simulink model "AuE6610_Project_CV"  (R2025a)
settings: Solver=ode4  StartTime=0.0  StopTime=1874  FixedStep=0.1  RelTol=1e-3
values from neighbouring files (symbols this model uses):
  area_frontal = 2.18    [CV_Powertrain.m]    (also in EV_Powertrain.m; database.m)
  curb_weight = 1377    [CV_Powertrain.m]    (also in EV_Powertrain.m; database.m)
  drag_coefficient = 0.29    [CV_Powertrain.m]    (also in EV_Powertrain.m; database.m)
  eng =     [Engine_Data.mat]
  fdr = 4.21    [CV_Powertrain.m]    (also in EV_Powertrain.m; database.m)
  fdr_inertia = 0.02    [CV_Powertrain.m]    (also in EV_Powertrain.m; database.m)
  gear = [3.54, 1.91, 1.31, 0.97, 0.71, 0.62]    [CV_Powertrain.m]    (also in EV_Powertrain.m = 1.5; database.m)
  gear_no = [1, 2, 3, 4, 5, 6]    [CV_Powertrain.m]    (also in EV_Powertrain.m = 1; database.m = [1,2,3,4,5,6])
  gear_selected = zeros(length(peddle_position), length(speed))    [CV_Powertrain.m]    (also in database.m = zeros(length(iso_power), length(speed)))
  idle_rpm = 500    [CV_Powertrain.m]    (also in EV_Powertrain.m = 1; database.m)
  max_engine_power = max((rpm_engine_data(1,:) * (pi/30)) .* torque_engine_data(end,:))    [CV_Powertrain.m]    (also in database.m = max((rpm_engine_data(1,:) * ( pi /30)) .* torque_engine_data)
  peddle_position = 0.1:0.05:1    [CV_Powertrain.m]    (also in database.m)
  radius = 0.4318    [CV_Powertrain.m]    (also in EV_Powertrain.m; database.m)
  redline_rpm = 6800    [CV_Powertrain.m]    (also in EV_Powertrain.m = 11000; database.m)
  rho_air = 1.18    [CV_Powertrain.m]    (also in EV_Powertrain.m = 1.21; database.m)
  rolling_resistance_coefficient = 0.01    [CV_Powertrain.m]    (also in EV_Powertrain.m; database.m)
  rpm_reference_array = rpm_engine_data(1,:)    [CV_Powertrain.m]    (also in database.m)
  speed = 0:1:52    [CV_Powertrain.m]    (also in database.m = 1:1:52)
  torque_engine_data = zeros(n_pressure_points, n_rpm_points)    [CV_Powertrain.m]    (also in database.m = zeros(length(vol_eff_intake_pressure_array),length(rpm)))
  torque_max = torque_engine_data(end,:)    [CV_Powertrain.m]    (also in database.m)
  trans_inertia = 0.04    [CV_Powertrain.m]    (also in EV_Powertrain.m; database.m)
  wheel_inertia = 0.95    [CV_Powertrain.m]    (also in EV_Powertrain.m; database.m)
libraries: slpidlib x1, simulink x1
settings Model: Creator=Qilun Zhu  LastModifiedBy=abhi
settings SolverCC: ZeroCrossAlgorithm=Adaptive  AlgebraicLoopSolver=TrustRegion
settings DataIOCC: ReturnWorkspaceOutputs=off
settings DebuggingCC: UnconnectedInputMsg=warning  UnconnectedOutputMsg=warning  UnconnectedLineMsg=warning  ArithmeticOperatorsInVariantConditions=warning
settings ModelReferenceCC: EnableRefExpFcnMdlSchedulingChecks=on
settings SFSimCC: SimUseLocalCustomCode=off  CustomCodeUndefinedFunction=UseInterfaceOnly
settings RTWCC: RTWUseLocalCustomCode=off  GPUComputeCapability=3.5  DLArmComputeVersion=19.05
settings CodeAppCC: StateflowObjectComments=on
settings SimscapeCC: SimscapeNormalizeSystem=off

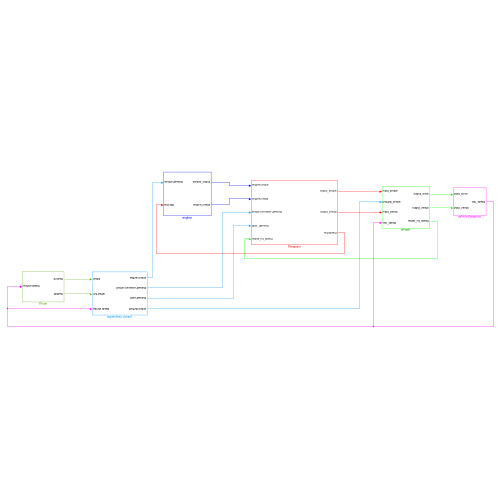
[thumbnail: Simulink's stored preview of the top-level diagram]
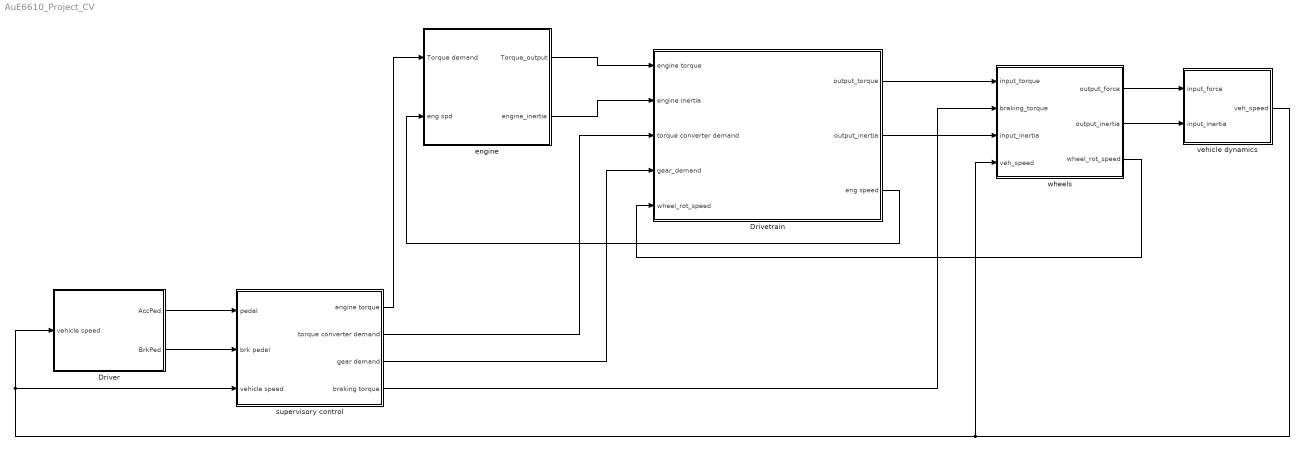
== system AuE6610_Project_CV ==
  Driver : Subsystem
  Drivetrain : Subsystem
  engine : Subsystem
  supervisory control : Subsystem
  vehicle dynamics : Subsystem
  wheels : Subsystem
  wires:
  supervisory control/1(engine torque) -> engine/1(Torque demand)
  wheels/1(output_force) -> vehicle dynamics/1(input_force)
  wheels/2(output_inertia) -> vehicle dynamics/2(input_inertia)
  supervisory control/4(braking torque) -> wheels/2(braking_torque)
  Driver/1(AccPed) -> supervisory control/1(" pedal")
  supervisory control/2(torque converter demand) -> Drivetrain/3(torque converter demand)
  supervisory control/3(gear demand) -> Drivetrain/4(gear_demand)
  engine/1(Torque_output) -> Drivetrain/1(engine torque)
  engine/2(engine_inertia) -> Drivetrain/2(engine inertia)
  wheels/3(wheel_rot_speed) -> Drivetrain/5(wheel_rot_speed)
  Drivetrain/1(output_torque) -> wheels/1(input_torque)
  Drivetrain/3(eng speed) -> engine/2(eng spd)
  Drivetrain/2(output_inertia) -> wheels/3(input_inertia)
  vehicle dynamics/1(veh_speed) -> Driver/1(vehicle speed), supervisory control/3(vehicle speed), wheels/4(veh_speed)
  Driver/2(BrkPed) -> supervisory control/2(" brk pedal")

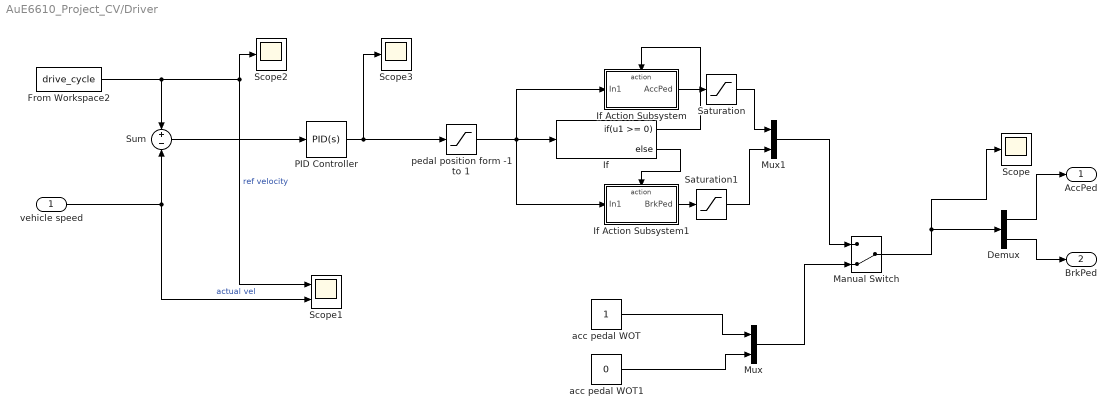
== system AuE6610_Project_CV/Driver ==
  vehicle speed : Inport
  Demux : Demux  Outputs=2
  From Workspace2 : FromWorkspace  VariableName=drive_cycle
  If : If  IfExpression=u1 >= 0
  If Action Subsystem : Subsystem  TreatAsAtomicUnit=on
  If Action Subsystem1 : Subsystem  TreatAsAtomicUnit=on
  Manual Switch : ManualSwitch  CurrentSetting=0
  Mux : Mux  Inputs=2
  Mux1 : Mux  Inputs=2
  PID Controller : slpidlib/PID Controller  Controller=PID  Form=Parallel  TimeDomain=Continuous-time  UseExternalTs=off  SampleTime=-1  IntegratorMethod=Forward Euler  FilterMethod=Forward Euler  ControllerParametersSource=internal  P=0.2  I=0.2  UseKiTs=off  D=0  UseExternalDerivativeSource=off  N=100  UseFilter=on  TunerSelectOption=Transfer Function Based (PID Tuner App)  InitialConditionSource=internal  InitialConditionForIntegrator=0  InitialConditionForFilter=0  DifferentiatorICPrevScaledInput=0  ExternalReset=none  TrackingMode=off  Kt=1  LimitOutput=off  SatLimitsSource=internal  UpperSaturationLimit=inf  LowerSaturationLimit=-inf  LinearizeAsGain=on  AntiWindupMode=none  Kb=1  LimitIntegrator=off  UpperIntegratorSaturationLimit=inf  LowerIntegratorSaturationLimit=-inf  POutMin=[]  POutMax=[]  IOutMin=[]  IOutMax=[]  DOutMin=[]  DOutMax=[]  NOutMin=[]  NOutMax=[]  SumOutMin=[]  SumOutMax=[]  SaturationOutMin=[]  SaturationOutMax=[]  PParamMin=[]  PParamMax=[]  IParamMin=[]  IParamMax=[]  DParamMin=[]  DParamMax=[]  NParamMin=[]  NParamMax=[]  KbParamMin=[]  KbParamMax=[]  KtParamMin=[]  KtParamMax=[]  KbOutMin=[]  KbOutMax=[]  KtOutMin=[]  KtOutMax=[]  IntegratorOutMin=[]  IntegratorOutMax=[]  FilterOutMin=[]  FilterOutMax=[]  SumI1OutMin=[]  SumI1OutMax=[]  SumI2OutMin=[]  SumI2OutMax=[]  SumI3OutMin=[]  SumI3OutMax=[]  SumI4OutMin=[]  SumI4OutMax=[]  SumDOutMin=[]  SumDOutMax=[]  DifferentiatorOutMin=[]  DifferentiatorOutMax=[]  FilterDiffOutCoefMin=[]  FilterDiffOutCoefMax=[]  ReciprocalOutMin=[]  ReciprocalOutMax=[]  SumDenOutMin=[]  SumDenOutMax=[]  SumNumOutMin=[]  SumNumOutMax=[]  DivideOutMin=[]  DivideOutMax=[]  UdiffTsProdOutMin=[]  UdiffTsProdOutMax=[]  NTsProdOutMin=[]  NTsProdOutMax=[]  UintegralTsProdOutMin=[]  UintegralTsProdOutMax=[]  UngainTsProdOutMin=[]  UngainTsProdOutMax=[]  ClampingZeroOutDataTypeStr=Inherit: Inherit via back propagation  ClampingZeroOutMin=[]  ClampingZeroOutMax=[]  FilterDenConstantOutDataTypeStr=Inherit: Inherit via back propagation  FilterDenConstantOutMin=[]  FilterDenConstantOutMax=[]  PCopyOutDataTypeStr=Inherit: Inherit via back propagation  PCopyOutMin=[]  PCopyOutMax=[]  NCopyOutDataTypeStr=Inherit: Inherit via back propagation  NCopyOutMin=[]  NCopyOutMax=[]  IntegratorContinuousStateAttributes=''  IntegratorStateMustResolveToSignalObject=off  IntegratorRTWStateStorageClass=Auto  FilterContinuousStateAttributes=''  FilterStateMustResolveToSignalObject=off  FilterRTWStateStorageClass=Auto  ParallelPVariant=InternalParameters  IdealPVariant=Disabled  IVariant=InternalParameters  DVariant=InternalParameters  IntegratorVariant=Continuous  SatVariant=Disabled  AWVariant=Passthrough  PCopyVariant=Disabled  TRVariant=Disabled  FdbkBlocksVariant=Forward  IdealPFdbkVariant=Disabled  SatFdbkVariant=Disabled  DerivativeFilterVariant=ContFilter  NVariant=InternalParameters  NCopyVariant=Disabled  FilterICVariant=InternalICsFilter  IntegratorICVariant=InternalICs  ExternalResetVariant=Disabled  TRSumVariant=Passthrough  SumFdbkVariant=Disabled  SumVariant=Sum_PID  TsampFilterVariant=InternalTs  TsampNgainVariant=Passthrough  TsampIntegralVariant=Disabled_SignalSpec  ExternalSaturationOutDataTypeStr=Inherit: Same as second input  DerivativeSourceVariant=ErrorSignal  PreIntVariant=InternalPreInt
  Saturation : Saturate  UpperLimit=1  LowerLimit=0
  Saturation1 : Saturate  UpperLimit=0  LowerLimit=-1
  Scope : Scope
      settings: ActiveDisplayYMinimum=-0.14734993314057482  ActiveDisplayYMaximum=0.25708356737728405
  Scope1 : Scope  NumInputPorts=2
      settings: ActiveDisplayYMinimum=-3.7898658117553516  ActiveDisplayYMaximum=28.746411818006802
  Scope2 : Scope
      settings: ActiveDisplayYMinimum=-1  ActiveDisplayYMaximum=1  DataLoggingVariableName=ScopeData2
  Scope3 : Scope
      settings: ActiveDisplayYMinimum=-1.9427647766660474  ActiveDisplayYMaximum=1.090909837606671  DataLoggingVariableName=ScopeData14
  Sum : Sum  Inputs=+-
  acc pedal WOT : Constant
  acc pedal WOT1 : Constant  Value=0
  pedal position form -1 to 1 : Saturate  UpperLimit=1  LowerLimit=-1  ZeroCross=off
  AccPed : Outport
  BrkPed : Outport  Port=2
  wires:
  Manual Switch/1 -> Demux/1, Scope/1
  If/1 -> If Action Subsystem/Action
  If/2 -> If Action Subsystem1/Action
  Sum/1 -> PID Controller/1
  pedal position form -1 to 1/1 -> If/1, If Action Subsystem1/1(In1), If Action Subsystem/1(In1)
  acc pedal WOT/1 -> Mux/1
  acc pedal WOT1/1 -> Mux/2
  Mux/1 -> Manual Switch/2
  Demux/1 -> AccPed/1
  Demux/2 -> BrkPed/1
  Mux1/1 -> Manual Switch/1
  From Workspace2/1 -> Scope2/1, Scope1/1, Sum/1  "ref velocity"
  vehicle speed/1 -> Scope1/2, Sum/2  "actual vel"
  PID Controller/1 -> Scope3/1, pedal position form -1 to 1/1
  If Action Subsystem/1(AccPed) -> Saturation/1
  Saturation/1 -> Mux1/1
  If Action Subsystem1/1(BrkPed) -> Saturation1/1
  Saturation1/1 -> Mux1/2

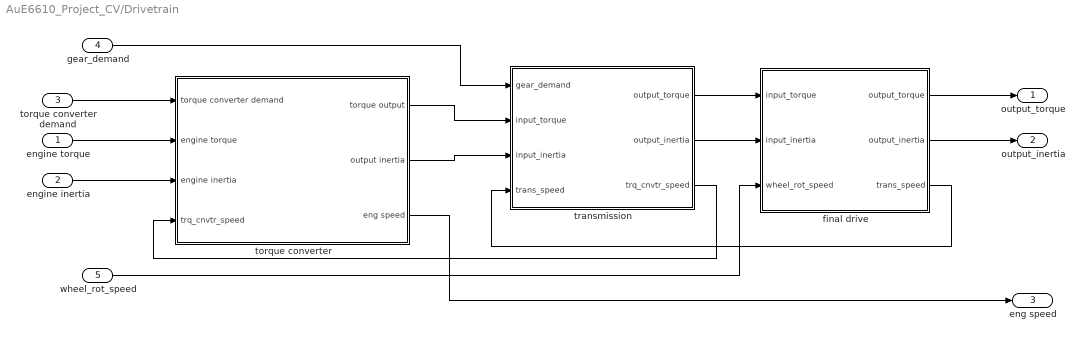
== system AuE6610_Project_CV/Drivetrain ==
  engine torque : Inport
  engine inertia : Inport  Port=2
  torque converter demand : Inport  Port=3
  gear_demand : Inport  Port=4
  wheel_rot_speed : Inport  Port=5
  final drive : Subsystem
      mask Display: image('C:\Users\bhatt\Desktop\driveline.jpg'); % Use "Edit Image" on toolstrip to change.
  torque converter : Subsystem
      mask Display: image('C:\Users\bhatt\Desktop\torque converter.jpg'); % Use "Edit Image" on toolstrip to change.
  transmission : Subsystem
      mask Display: image('C:\Users\bhatt\Desktop\gearbox.jpg'); % Use "Edit Image" on toolstrip to change.
  output_torque : Outport
  output_inertia : Outport  Port=2
  eng speed : Outport  Port=3
  wires:
  torque converter/3(eng speed) -> eng speed/1
  transmission/2(output_inertia) -> final drive/2(input_inertia)
  transmission/1(output_torque) -> final drive/1(input_torque)
  engine inertia/1 -> torque converter/3(engine inertia)
  torque converter/2(output inertia) -> transmission/3(input_inertia)
  final drive/3(trans_speed) -> transmission/4(trans_speed)
  torque converter/1(torque output) -> transmission/2(input_torque)
  transmission/3(trq_cnvtr_speed) -> torque converter/4(trq_cnvtr_speed)
  gear_demand/1 -> transmission/1(gear_demand)
  final drive/1(output_torque) -> output_torque/1
  engine torque/1 -> torque converter/2(engine torque)
  wheel_rot_speed/1 -> final drive/3(wheel_rot_speed)
  final drive/2(output_inertia) -> output_inertia/1
  torque converter demand/1 -> torque converter/1(torque converter demand)

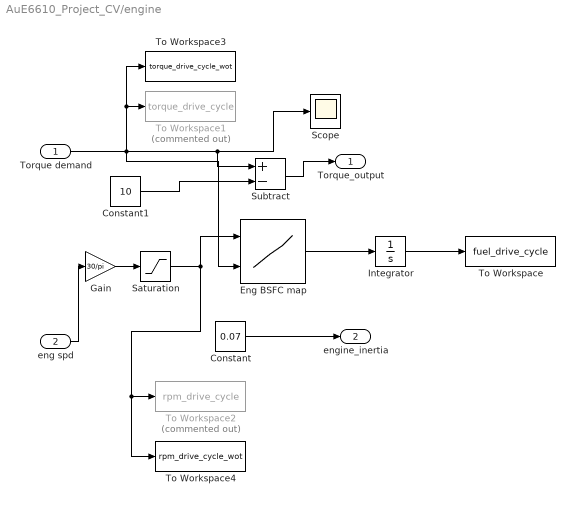
== system AuE6610_Project_CV/engine ==
  Torque demand : Inport
  eng spd : Inport  Port=2
  Constant : Constant  Value=0.07
  Constant1 : Constant  Value=10
  Eng BSFC map : Lookup_n-D  BreakpointsForDimension1=eng.BSFC.RPM  BreakpointsForDimension2=eng.BSFC.T  Table=eng.BSFC.fuel_rate  InternalRulePriority=Speed  RndMeth=Simplest
      settings: InputPortMap=u0,u1
  Gain : Gain  Gain=30/pi
  Integrator : Integrator
  Saturation : Saturate  UpperLimit=redline_rpm  LowerLimit=idle_rpm
  Scope : Scope
      settings: ActiveDisplayYMinimum=-16.725934018709687  ActiveDisplayYMaximum=150.53340616838722  DataLoggingVariableName=ScopeData3
  Subtract : Sum  Inputs=+-
  To Workspace : ToWorkspace  VariableName=fuel_drive_cycle  SampleTime=-1
  To Workspace1 : ToWorkspace  Commented=on  VariableName=torque_drive_cycle  SampleTime=-1
  To Workspace2 : ToWorkspace  Commented=on  VariableName=rpm_drive_cycle  SampleTime=-1
  To Workspace3 : ToWorkspace  VariableName=torque_drive_cycle_wot  SampleTime=-1
  To Workspace4 : ToWorkspace  VariableName=rpm_drive_cycle_wot  SampleTime=-1
  Torque_output : Outport
  engine_inertia : Outport  Port=2
  wires:
  eng spd/1 -> Gain/1
  Constant/1 -> engine_inertia/1
  Eng BSFC map/1 -> Integrator/1
  Torque demand/1 -> Subtract/1, Scope/1, To Workspace3/1, To Workspace1/1, Eng BSFC map/2
  Constant1/1 -> Subtract/2
  Subtract/1 -> Torque_output/1
  Gain/1 -> Saturation/1
  Saturation/1 -> To Workspace4/1, To Workspace2/1, Eng BSFC map/1
  Integrator/1 -> To Workspace/1

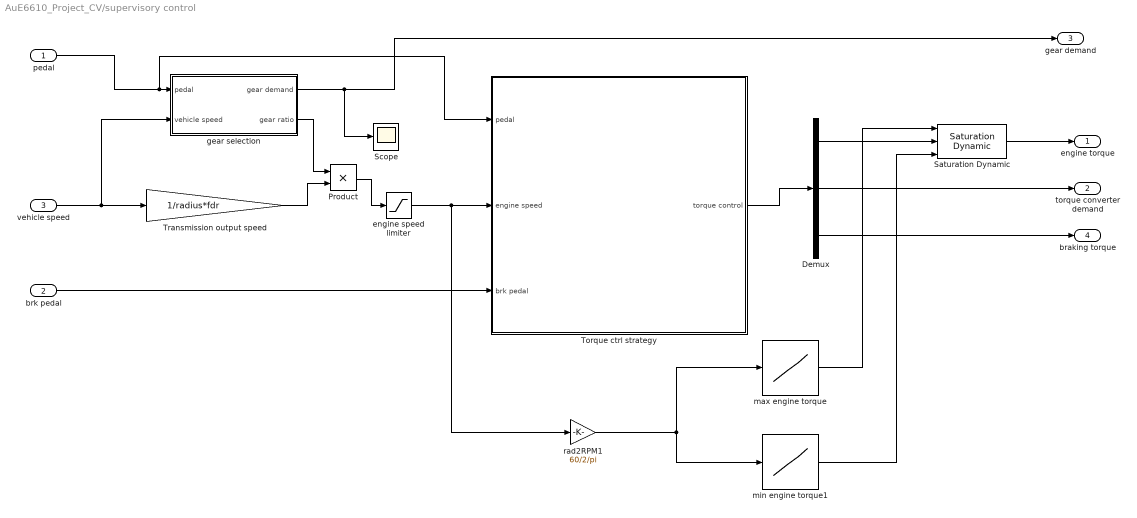
== system AuE6610_Project_CV/supervisory control ==
  " pedal" : Inport
  " brk pedal" : Inport  Port=2
  vehicle speed : Inport  Port=3
  Demux : Demux  Outputs=3
  Product : Product
  Saturation Dynamic : simulink/Discontinuities/Saturation Dynamic  OutMin=[]  OutMax=[]  OutDataTypeStr=Inherit: Same as second input  OutDataType=fixdt(1, 16)  OutScaling=2^-10  DoSatur=off
  Scope : Scope
      settings: ActiveDisplayYMinimum=-0.0099772185487898568  ActiveDisplayYMaximum=1.0167737074135261  DataLoggingVariableName=ScopeData16
  Torque ctrl strategy : Subsystem
  Transmission output speed : Gain  Gain=1/radius*fdr
  engine speed limiter : Saturate  UpperLimit=redline_rpm/60*2*pi  LowerLimit=idle_rpm/60*2*pi
  gear selection : Subsystem
  max engine torque : Lookup_n-D  NumberOfTableDimensions=1  BreakpointsForDimension1=rpm_reference_array  Table=torque_max  InternalRulePriority=Speed  RndMeth=Simplest
  min engine torque1 : Lookup_n-D  NumberOfTableDimensions=1  BreakpointsForDimension1=rpm_reference_array  Table=torque_engine_data(1,:)  InternalRulePriority=Speed  RndMeth=Simplest
  rad2RPM1 : Gain  Gain=60/2/pi
  engine torque : Outport
  torque converter demand : Outport  Port=2
  gear demand : Outport  Port=3
  braking torque : Outport  Port=4
  wires:
  max engine torque/1 -> Saturation Dynamic/1
  min engine torque1/1 -> Saturation Dynamic/3
  Demux/1 -> Saturation Dynamic/2
  Saturation Dynamic/1 -> engine torque/1
  Demux/2 -> torque converter demand/1
  Demux/3 -> braking torque/1
  Torque ctrl strategy/1(torque control) -> Demux/1
  rad2RPM1/1 -> max engine torque/1, min engine torque1/1
  engine speed limiter/1 -> rad2RPM1/1, Torque ctrl strategy/2(engine speed)
  Product/1 -> engine speed limiter/1
  " pedal"/1 -> Torque ctrl strategy/1(pedal), gear selection/1(pedal)
  vehicle speed/1 -> Transmission output speed/1, gear selection/2(vehicle speed)
  gear selection/2(gear ratio) -> Product/1
  Transmission output speed/1 -> Product/2
  gear selection/1(gear demand) -> Scope/1, gear demand/1
  " brk pedal"/1 -> Torque ctrl strategy/3(" brk pedal")

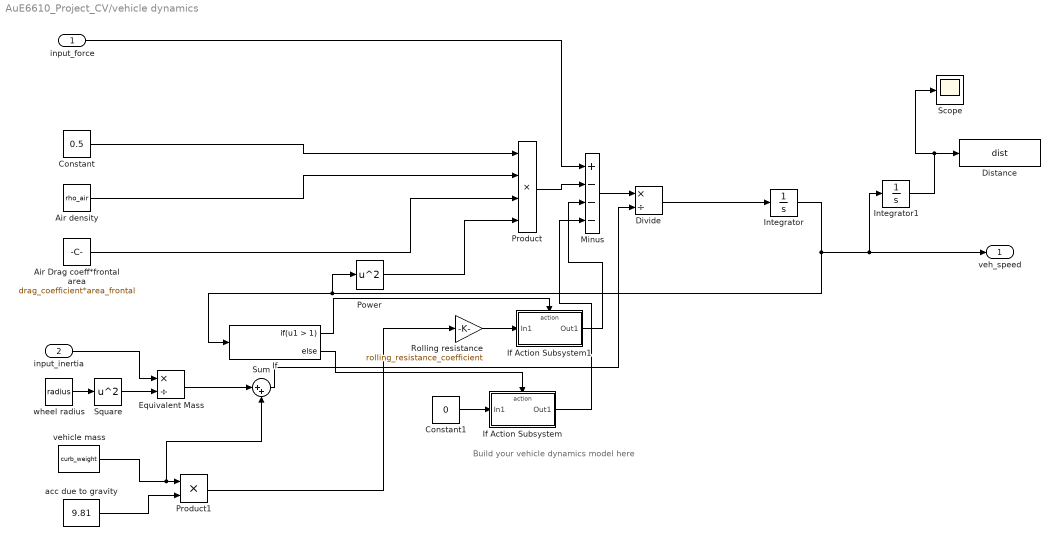
== system AuE6610_Project_CV/vehicle dynamics ==
  note: Build your vehicle dynamics model here
  input_force : Inport
  input_inertia : Inport  Port=2
  Air Drag coeff*frontal area : Constant  Value=drag_coefficient*area_frontal
  Air density : Constant  Value=rho_air
  Constant : Constant  Value=0.5
  Constant1 : Constant  Value=0
  Distance : ToWorkspace  VariableName=dist  SampleTime=-1
      settings: Save2DSignal=2-D array (concatenate along first dimension)
  Divide : Product  Inputs=*/
  Equivalent Mass : Product  Inputs=*/
  If : If  IfExpression=u1 > 1
  If Action Subsystem : Subsystem  TreatAsAtomicUnit=on
  If Action Subsystem1 : Subsystem  TreatAsAtomicUnit=on
  Integrator : Integrator
  Integrator1 : Integrator
  Minus : Sum  Inputs=+---
  Power : Math  Operator=square
  Product : Product  Inputs=4
  Product1 : Product
  "Rolling resistance " : Gain  Gain=rolling_resistance_coefficient
  Scope : Scope
      settings: ActiveDisplayYMinimum=-2221.2760263403779  ActiveDisplayYMaximum=19991.484237063407  DataLoggingVariableName=ScopeData5
  Square : Math  Operator=square
  Sum : Sum  Inputs=|++
  acc due to gravity : Constant  Value=9.81
  vehicle mass : Constant  Value=curb_weight
  wheel radius : Constant  Value=radius
  veh_speed : Outport
  wires:
  Product/1 -> Minus/2
  Integrator/1 -> If/1, Power/1, Integrator1/1, veh_speed/1
  If/1 -> If Action Subsystem1/Action
  If Action Subsystem1/1(Out1) -> Minus/3
  Divide/1 -> Integrator/1
  If Action Subsystem/1(Out1) -> Minus/4
  Minus/1 -> Divide/1
  "Rolling resistance "/1 -> If Action Subsystem1/1(In1)
  If/2 -> If Action Subsystem/Action
  input_force/1 -> Minus/1
  Constant/1 -> Product/1
  Air density/1 -> Product/2
  Air Drag coeff*frontal area/1 -> Product/3
  Power/1 -> Product/4
  vehicle mass/1 -> Sum/2, Product1/1
  acc due to gravity/1 -> Product1/2
  Product1/1 -> "Rolling resistance "/1
  Constant1/1 -> If Action Subsystem/1(In1)
  wheel radius/1 -> Square/1
  Square/1 -> Equivalent Mass/2
  input_inertia/1 -> Equivalent Mass/1
  Equivalent Mass/1 -> Sum/1
  Sum/1 -> Divide/2
  Integrator1/1 -> Scope/1, Distance/1

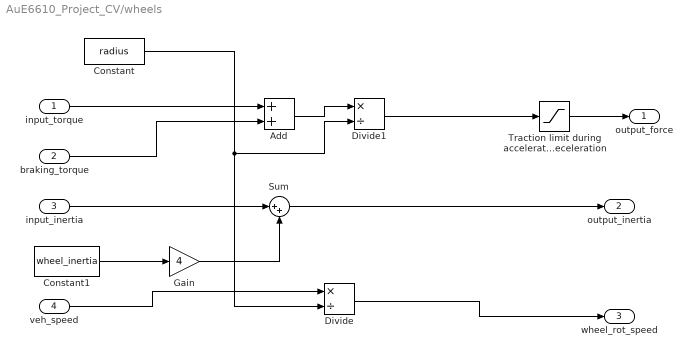
== system AuE6610_Project_CV/wheels ==
  input_torque : Inport
  braking_torque : Inport  Port=2
  input_inertia : Inport  Port=3
  veh_speed : Inport  Port=4
  Add : Sum
  Constant : Constant  Value=radius
  Constant1 : Constant  Value=wheel_inertia
  Divide : Product  Inputs=*/
  Divide1 : Product  Inputs=*/
  Gain : Gain  Gain=4
  Sum : Sum  Inputs=|++
  Traction limit during acceleration or deceleration : Saturate  UpperLimit=9740.781  LowerLimit=-9740.781
  output_force : Outport
  output_inertia : Outport  Port=2
  wheel_rot_speed : Outport  Port=3
  wires:
  Traction limit during acceleration or deceleration/1 -> output_force/1
  Constant/1 -> Divide1/2, Divide/2
  veh_speed/1 -> Divide/1
  Divide/1 -> wheel_rot_speed/1
  Constant1/1 -> Gain/1
  input_inertia/1 -> Sum/1
  Gain/1 -> Sum/2
  Sum/1 -> output_inertia/1
  input_torque/1 -> Add/1
  braking_torque/1 -> Add/2
  Add/1 -> Divide1/1
  Divide1/1 -> Traction limit during acceleration or deceleration/1

== system AuE6610_Project_CV/Driver/If Action Subsystem ==
  In1 : Inport
  Action Port : ActionPort  ActionPortLabel=if(u1 >= 0)
  AccPed : Outport
  wires:
  In1/1 -> AccPed/1

== system AuE6610_Project_CV/Driver/If Action Subsystem1 ==
  In1 : Inport
  Action Port : ActionPort  ActionPortLabel=else
  BrkPed : Outport
  wires:
  In1/1 -> BrkPed/1

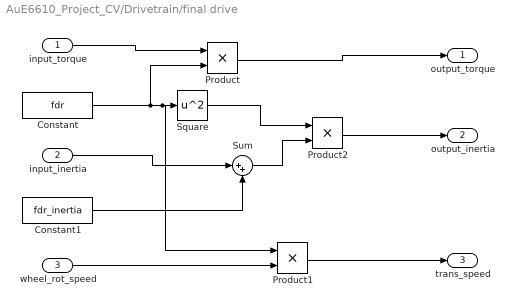
== system AuE6610_Project_CV/Drivetrain/final drive ==
  input_torque : Inport
  input_inertia : Inport  Port=2
  wheel_rot_speed : Inport  Port=3
  Constant : Constant  Value=fdr
  Constant1 : Constant  Value=fdr_inertia
  Product : Product
  Product1 : Product
  Product2 : Product
  Square : Math  Operator=square
  Sum : Sum  Inputs=|++
  output_torque : Outport
  output_inertia : Outport  Port=2
  trans_speed : Outport  Port=3
  wires:
  input_torque/1 -> Product/1
  Constant/1 -> Square/1, Product1/1, Product/2
  Product/1 -> output_torque/1
  input_inertia/1 -> Sum/1
  Constant1/1 -> Sum/2
  wheel_rot_speed/1 -> Product1/2
  Product1/1 -> trans_speed/1
  Product2/1 -> output_inertia/1
  Sum/1 -> Product2/2
  Square/1 -> Product2/1

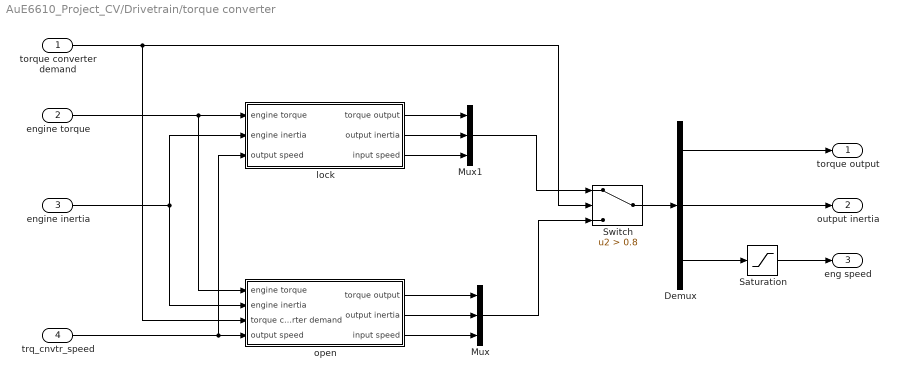
== system AuE6610_Project_CV/Drivetrain/torque converter ==
  torque converter demand : Inport
  engine torque : Inport  Port=2
  engine inertia : Inport  Port=3
  trq_cnvtr_speed : Inport  Port=4
  Demux : Demux  Outputs=3
  Mux : Mux  Inputs=3
  Mux1 : Mux  Inputs=3
  Saturation : Saturate  UpperLimit=6800/60*2*pi  LowerLimit=500/60*2*pi
  Switch : Switch  Criteria=u2 > Threshold  Threshold=0.8  SaturateOnIntegerOverflow=off  InputSameDT=off
  lock : Subsystem
  open : Subsystem
  torque output : Outport
  output inertia : Outport  Port=2
  eng speed : Outport  Port=3
  wires:
  engine torque/1 -> open/1(engine torque), lock/1(engine torque)
  engine inertia/1 -> open/2(engine inertia), lock/2(engine inertia)
  trq_cnvtr_speed/1 -> open/4(output speed), lock/3(output speed)
  open/1(torque output) -> Mux/1
  open/2(output inertia) -> Mux/2
  open/3(input speed) -> Mux/3
  lock/2(output inertia) -> Mux1/2
  lock/1(torque output) -> Mux1/1
  lock/3(input speed) -> Mux1/3
  torque converter demand/1 -> Switch/2, open/3(torque converter demand)
  Mux1/1 -> Switch/1
  Mux/1 -> Switch/3
  Switch/1 -> Demux/1
  Demux/1 -> torque output/1
  Demux/2 -> output inertia/1
  Demux/3 -> Saturation/1
  Saturation/1 -> eng speed/1

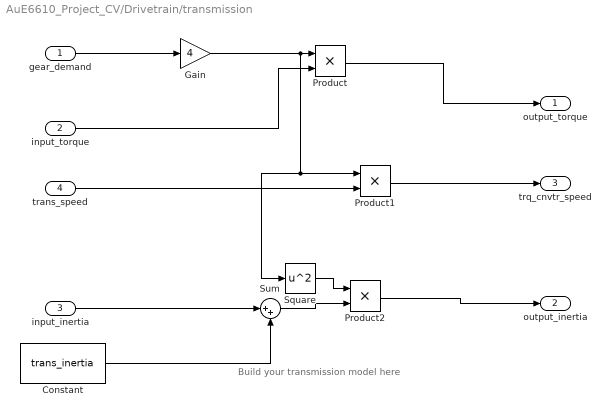
== system AuE6610_Project_CV/Drivetrain/transmission ==
  note: Build your transmission model here
  gear_demand : Inport
  input_torque : Inport  Port=2
  input_inertia : Inport  Port=3
  trans_speed : Inport  Port=4
  Constant : Constant  Value=trans_inertia
  Gain : Gain  Gain=4
  Product : Product
  Product1 : Product
  Product2 : Product
  Square : Math  Operator=square
  Sum : Sum  Inputs=|++
  output_torque : Outport
  output_inertia : Outport  Port=2
  trq_cnvtr_speed : Outport  Port=3
  wires:
  gear_demand/1 -> Gain/1
  Gain/1 -> Product1/1, Square/1, Product/1
  input_torque/1 -> Product/2
  Product/1 -> output_torque/1
  Constant/1 -> Sum/2
  input_inertia/1 -> Sum/1
  trans_speed/1 -> Product1/2
  Product1/1 -> trq_cnvtr_speed/1
  Square/1 -> Product2/1
  Sum/1 -> Product2/2
  Product2/1 -> output_inertia/1

== system AuE6610_Project_CV/supervisory control/Torque ctrl strategy ==
  pedal : Inport
  engine speed : Inport  Port=2
  " brk pedal" : Inport  Port=3
  Mux : Mux  Inputs=3
  Mux1 : Mux  Inputs=3
  Switch : Switch  Criteria=u2 > Threshold  ZeroCross=off  SaturateOnIntegerOverflow=off  InputSameDT=off
  accelerating : Subsystem
  decelerating : Subsystem
  torque control : Outport
  wires:
  engine speed/1 -> accelerating/2(engine speed), decelerating/1(engine speed)
  accelerating/1(engine torque) -> Mux/1
  accelerating/2(torque converter demand) -> Mux/2
  accelerating/3(braking torque) -> Mux/3
  decelerating/3(braking torque) -> Mux1/3
  decelerating/2(torque converter demand) -> Mux1/2
  decelerating/1(engine torque) -> Mux1/1
  Mux/1 -> Switch/1
  Mux1/1 -> Switch/3
  pedal/1 -> Switch/2, accelerating/1(acc pedal)
  Switch/1 -> torque control/1
  " brk pedal"/1 -> decelerating/2(brk pedal)

== system AuE6610_Project_CV/supervisory control/gear selection ==
  pedal : Inport
  vehicle speed : Inport  Port=2
  Maximum_Engine_Power : Constant  Commented=on  Value=max_engine_power
  gear map : Lookup_n-D  BreakpointsForDimension1=peddle_position  BreakpointsForDimension2=speed  Table=gear_selected  InterpMethod=Flat  InternalRulePriority=Speed  RndMeth=Simplest
      settings: InputPortMap=u0,u1
  selected gear ratio : Lookup_n-D  NumberOfTableDimensions=1  BreakpointsForDimension1=gear_no  Table=gear  InterpMethod=Flat  InternalRulePriority=Speed  RndMeth=Simplest
  gear demand : Outport
  gear ratio : Outport  Port=2
  wires:
  vehicle speed/1 -> gear map/2
  pedal/1 -> gear map/1
  gear map/1 -> gear demand/1, selected gear ratio/1
  selected gear ratio/1 -> gear ratio/1

== system AuE6610_Project_CV/vehicle dynamics/If Action Subsystem ==
  In1 : Inport
  Action Port : ActionPort  ActionPortLabel=else
  Out1 : Outport
  wires:
  In1/1 -> Out1/1

== system AuE6610_Project_CV/vehicle dynamics/If Action Subsystem1 ==
  In1 : Inport
  Action Port : ActionPort  ActionPortLabel=if(u1 > 1)
  Out1 : Outport
  wires:
  In1/1 -> Out1/1

== system AuE6610_Project_CV/Drivetrain/torque converter/lock ==
  engine torque : Inport
  engine inertia : Inport  Port=2
  output speed : Inport  Port=3
  torque output : Outport
  output inertia : Outport  Port=2
  input speed : Outport  Port=3
  wires:
  output speed/1 -> input speed/1
  engine torque/1 -> torque output/1
  engine inertia/1 -> output inertia/1

== system AuE6610_Project_CV/Drivetrain/torque converter/open ==
  engine torque : Inport
  engine inertia : Inport  Port=2
  torque converter demand : Inport  Port=3
  output speed : Inport  Port=4
  Constant : Constant  Value=0
  Constant1 : Constant  Value=0
  Divide : Product  Inputs=*/
  Integrator : Integrator  ExternalReset=falling  InitialConditionSource=external  InitialCondition=eng.rpm_idle/60*2*pi  ZeroCross=off
  torque output : Outport
  output inertia : Outport  Port=2
  input speed : Outport  Port=3
  wires:
  Constant/1 -> torque output/1
  engine torque/1 -> Divide/1
  engine inertia/1 -> Divide/2
  Divide/1 -> Integrator/1
  Integrator/1 -> input speed/1
  Constant1/1 -> output inertia/1
  torque converter demand/1 -> Integrator/2
  output speed/1 -> Integrator/3

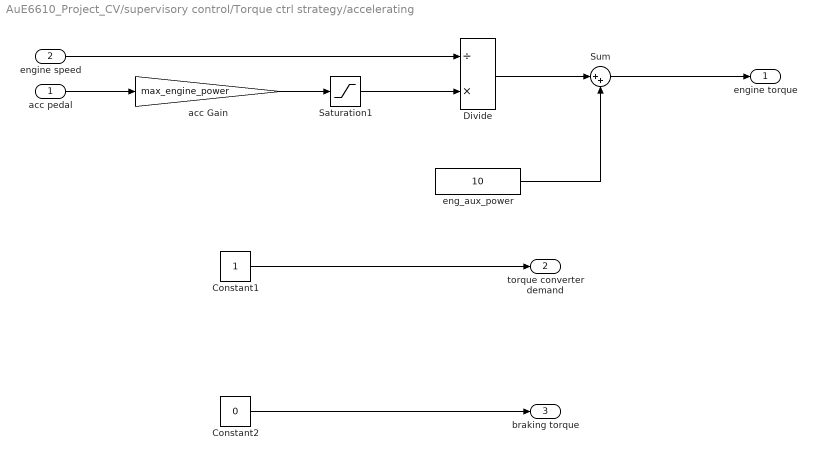
== system AuE6610_Project_CV/supervisory control/Torque ctrl strategy/accelerating ==
  acc pedal : Inport
  engine speed : Inport  Port=2
  Constant1 : Constant
  Constant2 : Constant  Value=0
  Divide : Product  Inputs=/*
  Saturation1 : Saturate  UpperLimit=max_engine_power  LowerLimit=0  ZeroCross=off
  Sum : Sum  Inputs=|++
  acc Gain : Gain  Gain=max_engine_power
  eng_aux_power : Constant  Value=10
  engine torque : Outport
  torque converter demand : Outport  Port=2
  braking torque : Outport  Port=3
  wires:
  engine speed/1 -> Divide/1
  eng_aux_power/1 -> Sum/2
  Divide/1 -> Sum/1
  Sum/1 -> engine torque/1
  Constant1/1 -> torque converter demand/1
  Constant2/1 -> braking torque/1
  acc Gain/1 -> Saturation1/1
  acc pedal/1 -> acc Gain/1
  Saturation1/1 -> Divide/2

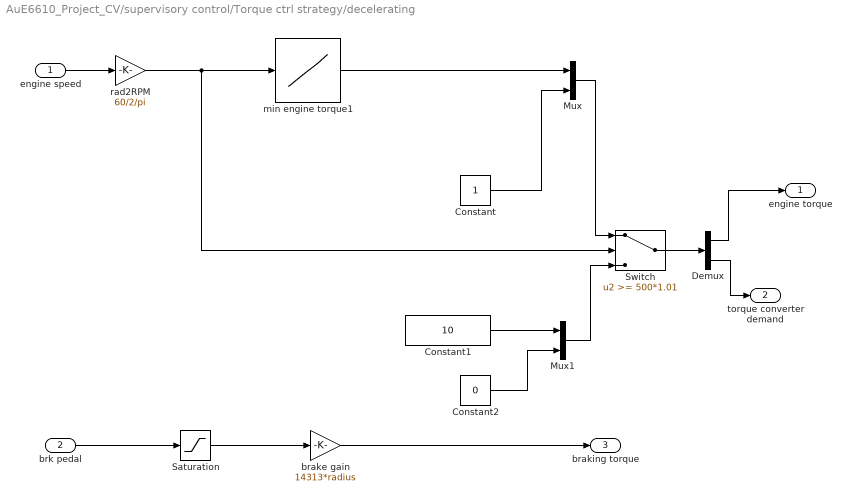
== system AuE6610_Project_CV/supervisory control/Torque ctrl strategy/decelerating ==
  engine speed : Inport
  brk pedal : Inport  Port=2
  Constant : Constant
  Constant1 : Constant  Value=10
  Constant2 : Constant  Value=0
  Demux : Demux  Outputs=2
  Mux : Mux  Inputs=2
  Mux1 : Mux  Inputs=2
  Saturation : Saturate  UpperLimit=0  LowerLimit=-1
  Switch : Switch  Threshold=500*1.01  ZeroCross=off  SaturateOnIntegerOverflow=off  InputSameDT=off
  brake gain : Gain  Gain=14313*radius
  min engine torque1 : Lookup_n-D  NumberOfTableDimensions=1  BreakpointsForDimension1=eng.T_max.RPM  Table=eng.T_min.T_min  InternalRulePriority=Speed  RndMeth=Simplest
  rad2RPM : Gain  Gain=60/2/pi
  engine torque : Outport
  torque converter demand : Outport  Port=2
  braking torque : Outport  Port=3
  wires:
  engine speed/1 -> rad2RPM/1
  rad2RPM/1 -> Switch/2, min engine torque1/1
  min engine torque1/1 -> Mux/1
  Constant/1 -> Mux/2
  Mux/1 -> Switch/1
  Constant1/1 -> Mux1/1
  Constant2/1 -> Mux1/2
  Mux1/1 -> Switch/3
  Switch/1 -> Demux/1
  Demux/1 -> engine torque/1
  Demux/2 -> torque converter demand/1
  brk pedal/1 -> Saturation/1
  brake gain/1 -> braking torque/1
  Saturation/1 -> brake gain/1
